simulink model "rgyro"  (Simulink 5.0)
settings: Solver=ode45  StartTime=0.0  StopTime=2  RelTol=1e-3

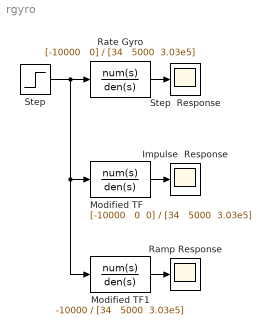
== system rgyro ==
  Impulse  Response : Scope
      settings: SaveName=imp  DataFormat=Array
  Modified TF : TransferFcn  Numerator="[-10000   0  0]"  Denominator="[34   5000  3.03e5]"
  Modified TF1 : TransferFcn  Numerator=-10000  Denominator="[34   5000  3.03e5]"
  Ramp Response : Scope
      settings: SaveName=ramp  DataFormat=Array
  Rate Gyro : TransferFcn  Numerator="[-10000   0]"  Denominator="[34   5000  3.03e5]"
  Step : Step  Time=0.1  After=0.1  SampleTime=0
  Step  Response : Scope
      settings: SaveName=step  DataFormat=Array
  wires:
  Step/1 -> Rate Gyro/1, Modified TF/1, Modified TF1/1
  Rate Gyro/1 -> Step  Response/1
  Modified TF/1 -> Impulse  Response/1
  Modified TF1/1 -> Ramp Response/1
